simulink model "tristezaydolor"  (R2021a)
settings: Solver=VariableStepAuto  StartTime=0.0  StopTime=5  RelTol=1e-3
values from neighbouring files (symbols this model uses):
  A_d = I + A*Ts    [observador_completo.m]
  B_d = B*Ts    [observador_completo.m]
  C = [ 1  0  0  0 ... (first row only)    [observador_completo.m]
  C_d = C    [observador_completo.m]
undefined symbols (not defined in the file or in its folder): A_obs, B_obs, C_d2
libraries: dspsrcs4 x1
settings Model: Creator=amali  LastModifiedBy=mogic

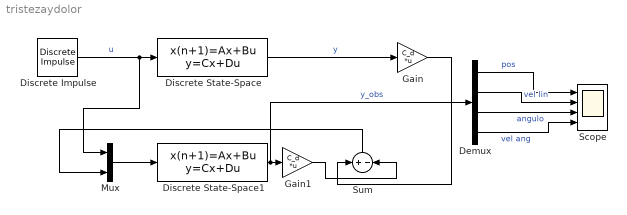
== system tristezaydolor ==
  Demux : Demux
  Discrete Impulse : dspsrcs4/Discrete  Impulse  Delay=0  SampleTime=1  FrameSample=1  OutputFrames=off  dataType=double  isSigned=on  wordLen=16  udDataType=sfix(16)  fracBitsMode=Best precision  numFracBits=15  OutDataTypeStr=double  LastOutDataTypeStr=double
  Discrete State-Space : DiscreteStateSpace  A=A_d  B=B_d  C=C  D=[0;0]  SampleTime=0.02
  Discrete State-Space1 : DiscreteStateSpace  A=A_obs  B=B_obs  C=C_d2  D=zeros(4,3)  SampleTime=0.02
  Gain : Gain  Gain=C_d  Multiplication=Matrix(K*u)
  Gain1 : Gain  Gain=C_d  Multiplication=Matrix(K*u)
  Mux : Mux  Inputs=2
  Scope : Scope  NumInputPorts=4
  Sum : Sum  Inputs=+|-
  wires:
  Discrete State-Space/1 -> Gain/1  "y"
  Gain/1 -> Sum/1
  Discrete Impulse/1 -> Mux/1, Discrete State-Space/1  "u"
  Discrete State-Space1/1 -> Demux/1, Gain1/1  "y_obs"
  Mux/1 -> Discrete State-Space1/1
  Sum/1 -> Mux/2
  Gain1/1 -> Sum/2
  Demux/2 -> Scope/2  "vel lin"
  Demux/1 -> Scope/1  "pos"
  Demux/3 -> Scope/3  "angulo"
  Demux/4 -> Scope/4  "vel ang"
